simulink library "qss_tb_library"  (Simulink 10.0)
settings: Solver=ode45  StartTime=0.0  StopTime=1220  RelTol=1e-3
undefined symbols (not defined in the file): automatic_gearbox, cc_done, delta_h_C_air, DiscIntNeverNeededParam, dw_GG_c, eta_EG_map, eta_EM_map, eta_ice, g, h, H_o_m, H_u, i_FC_in, i_FC_max, k1, k2, k3, k4, k_cs, M_air, manual_gearbox, P_aux, P_CE_cutoff, P_CE_idle, P_CE_recup, P_CVT_opt, Q_BT_min, Q_SC_IC, r, rho, rho_f, t_c, T_CE_cutoff, T_CE_max, T_EG_c, T_EG_max, T_EM_max, theta_CE, theta_EM, V_CE_map, V_FC_out, w_CE_idle, w_CE_max, w_CE_upper, w_CVT_opt, w_EG_row, w_EG_upper, w_EM_row, w_EM_upper, w_GG_c
(part 1 of 4)
settings Model: Creator=buehli  LastModifiedBy=barka  ModifiedComment=rickardarvidsson -- Wed Jul 11 10:39:34 2018 -- Version 1.277  ExtModeAutoUpdateStatusClock=off
settings Model: ModifiedHistory=|
  | rickardarvidsson -- Wed Jul 11 10:39:34 2018 -- Version 1.277
  | 
  | rickardarvidsson -- Wed Jul 11 10:39:34 2018 -- Version 1.277
  | 
  | rickardarvidsson -- Wed Jul 11 10:39:21 2018 -- Version 1.276
  | 
  | rickardarvidsson -- Wed Jul 11 10:39:08 2018 -- Version 1.275
  | 
  | 2018b:
  | Updated Energy Buffer Libraries with 48V, HEV, PHEV, BEV Batteries.
  | Resistance, energy and current values adjusted for each cell type

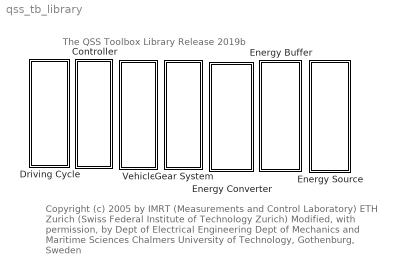
== system qss_tb_library ==
  note: Copyright (c) 2005 by IMRT (Measurements and Control Laboratory)
      | ETH Zurich (Swiss Federal Institute of Technology Zurich)
      |
      | Modified, with permission, by
      | Dept of Electrical Engineering
      | Dept of Mechanics and Maritime Sciences
      | Chalmers University of Technology, Gothenburg, Sweden
  note: The QSS Toolbox Library Release 2019b
  Controller : Subsystem
      mask Display: disp('Controller')
  Driving Cycle : Subsystem
      mask Display: disp('Driving Cycle')
  Energy Buffer : Subsystem
      mask Display: disp('Energy Buffer')
  Energy Converter : Subsystem
      mask Display: disp('Energy Converter')
  Energy Source : Subsystem
      mask Display: disp('Energy Source')
  Gear System : Subsystem
      mask Display: disp('Gear System')
  Vehicle : Subsystem
      mask Display: disp('Vehicle')

== system qss_tb_library/Controller ==
  Battery Controller : Subsystem  mask(Battery Controller){}
      mask help:
      | Control strategy (very primitive):
      | ========================
      | As soon as battery charge drops below level Q_BT_min, the CE/Generator
      | are started and operated at given load/speed for a fixed time period.
      | This time has been selected to guarantee the same battery level at the
      | end of the cycle.
      mask init:
      | init_BT_ctrl;
  CVT Controller : Subsystem  Tag=cvt controller  mask(CVT Controller){j_CVT_min=3, j_CVT_max=15, w_wheel_min=3, w_CVT_idle=100, w_CVT_upper=300}
      mask prompts: j_CVT_min "Lower gear ratio limit [-]"; j_CVT_max "Upper gear ratio limit [-]"; w_wheel_min "Minimum wheel speed [rad/s]"; w_CVT_idle "CVT idle speed [rad/s]"; w_CVT_upper "Maximum CVT speed [rad/s]"
      mask help:
      | This block calculates the optimum gear ratio and its change during one integration step for a CVT.
      |
      | Input:
      | =====
      | 	v	Speed [m/s]
      | 	dv_dt	Acceleration [m/s^2]
      |
      | Output:
      | ======
      | 	v_delay	Speed one step delayed [m/s]
      | 	dv_dt_delay	Acceleration one step delayed [m/s^2]
      | 	j_CVT	Gear ratio [-]
      | 	dj_CVT	Change of gear ratio [1/s]
      mask init:
      | init_CVT_ctrl;
  Control Unit (empty template) : Subsystem  Tag=control unit  mask(Control Unit){}
      mask help:
      | This block gives the user the opportunity to design his/her own control unit.
      |
      | The user can define the inputs and outputs  by himself/herself.
  "Hybrid Controller Unit  (Parallel, empty)" : Subsystem  mask(Hybrid Controller Unit){}
      mask help: Design your control strategy in this block.
      mask init:
      | init_HCU_parallel;

== system qss_tb_library/Driving Cycle ==
  Driving Cycle : Subsystem  Tag=cycle  mask(Driving Cycle){cyclename1=NEDC, stepsize=1, autostop=on}
      mask prompts: cyclename1 "Choose a cycle"; stepsize "Step size [s]"; autostop "Enable automatic simulation stop"
      mask help:
      | This block loads the cycle data such as time, speed, acceleration and gear number,  from the specified data file and makes it available on the output of the cycle block.
      |
      | Output:
      | ======
      | 	v	Speed [m/s]
      | 	a	Acceleration [m/s^2]
      | 	i	Gear number [-]
      | 	x_tot	Total distance [m]
      |
      | Tip:
      | ===
      | Probably you don't need the gear number "i". If so you can terminate
      | it with a "Terminator" out of the "Simulink Library/Connections."
      |
      | Driving cycle:
      | ===
      | Select a driving cycle from the list below or specify your own (place your .mat file in the
      | directory Data/DrivingCycles/UserDefined)
      |
      | ECE_MAN
      | ECE_R15s
      | EUDC
      | EUDC_MAN
      | City
      | City_MAN
      | NEDC
      | NEDC_MANl
      | GOT1
      | GOT2
      | GOT3
      | 10_15_MODE
      | 10_MODE
      | 10_MODE_3
      | 11_MODE
      | 11_MODE_4
      | 15_MODE
      | City_I
      | City_II
      | FTP_75
      | FTP_Highway
      |
      | WLTC
      | RTS95
      |
      |
      | Step size:
      | ========
      | Default value is 1. Don't change it, unless you are familiar with the programs of the QSS TB.
      |
      | Enable automatic simulation stop:
      | ===========================
      | Stops the simulation automatically at the end of the cycle.
      | Be careful: If you have a component in your model that has to run after the cycle has finished, e.g. a battery to charge, remove the mark!
      mask init:
      | init_driving_cycle1;
      mask Display: plot(T_zplot, V_zplot);
  Driving Cycle  (with performance  test possibility) : Subsystem  Tag=cycle  mask(Driving Cycle){cyclenr=Europe: NEDC, stepsize=1, autostop=on, test=off, v_init=0, v_end=0, acc_constant=0, gearon=[10 25 40 70], gearoff=[5 15 30 50]}
      mask prompts: cyclenr "Choose a cycle"; stepsize "Step size [s]"; autostop "Enable automatic simulation stop"; test "Acceleration performance test"; v_init "Start velocity [km/h]"; v_end "End velocity [km/h]"; acc_constant "Constant acceleration [m/s2]"; gearon "Switching points for upshift [km/h]"; gearoff "Switching points for downshift [km/h]"
      mask help:
      | This block loads the cycle data such as time, speed, acceleration and gear number,  from the specified data file and makes it available on the output of the cycle block.
      |
      | Output:
      | ======
      | 	v	Speed [m/s]
      | 	a	Acceleration [m/s^2]
      | 	i	Gear number [-]
      | 	x_tot	Total distance [m]
      |
      | Tip:
      | ===
      | Probably you don't need the gear number "i". If so you can terminate
      | it with a "Terminator" out of the "Simulink Library/Connections."
      |
      | Step size:
      | ========
      | Default value is 1. Don't change it, unless you are familiar with the programs of the QSS TB.
      |
      | Enable automatic simulation stop:
      | ===========================
      | Stops the simulation automatically at the end of the cycle.
      | Be careful: If you have a component in your model that has to run after the cycle has finished, e.g. a battery to charge, remove the mark!
      |
      | Acceleration Performance Test:
      | ===========================
      | This option will perform an acceleration test using a constant acceleration, from
      | start velocity to end velocity.
      | Gear shifting occuring to shifting schedule, defined by the user.
      mask init:
      | init_driving_cycle;
      mask TypeOptions cyclenr: Europe: ECE manual | Europe: ECE R15 spez | Europe: ECE R15 | Europe: EUDC | Europe: EUDC manual | Europe: City | Europe: City manual | Europe: NEDC | Europe: NEDC manual | Europe: GOT1 | Europe: GOT2 | Europe: GOT3 | Japan:  10-15-Mode | Japan:  10-Mode | Japan:  10-Mode-3 | Japan:  11-Mode | Japan:  11-Mode-4 | Japan:  15-Mode | USA:    City-I | USA:    City-II | USA:    FTP-75 | USA:    FTP-Highway
      mask Display: plot(T_zplot, V_zplot);
  Driving Cycle (no gradient) : Subsystem  Tag=cycle  mask(Driving Cycle){cyclename1=NEDC, stepsize=1, autostop=on}
      mask prompts: cyclename1 "Choose a cycle"; stepsize "Step size [s]"; autostop "Enable automatic simulation stop"
      mask help:
      | This block loads the cycle data such as time, speed, acceleration and gear number,  from the specified data file and makes it available on the output of the cycle block.
      |
      | Output:
      | ======
      | 	v	Speed [m/s]
      | 	a	Acceleration [m/s^2]
      | 	i	Gear number [-]
      | 	x_tot	Total distance [m]
      |
      | Tip:
      | ===
      | Probably you don't need the gear number "i". If so you can terminate
      | it with a "Terminator" out of the "Simulink Library/Connections."
      |
      | Driving cycle:
      | ===
      | Select a driving cycle from the list below or specify your own (place your .mat file in the
      | directory Data/DrivingCycles/UserDefined)
      |
      | ECE_MAN
      | ECE_R15s
      | EUDC
      | EUDC_MAN
      | City
      | City_MAN
      | NEDC
      | NEDC_MANl
      | GOT1
      | GOT2
      | GOT3
      | 10_15_MODE
      | 10_MODE
      | 10_MODE_3
      | 11_MODE
      | 11_MODE_4
      | 15_MODE
      | City_I
      | City_II
      | FTP_75
      | FTP_Highway
      |
      |
      | Step size:
      | ========
      | Default value is 1. Don't change it, unless you are familiar with the programs of the QSS TB.
      |
      | Enable automatic simulation stop:
      | ===========================
      | Stops the simulation automatically at the end of the cycle.
      | Be careful: If you have a component in your model that has to run after the cycle has finished, e.g. a battery to charge, remove the mark!
      mask init:
      | init_driving_cycle1;
      mask Display: plot(T_zplot, V_zplot);

== system qss_tb_library/Energy Buffer ==
  note: Batteries for hybrid vehicles
  48V Battery : Subsystem  Tag=battery  mask(Battery){cell_series=14, cell_parallel=1, Q_BT_IC_rel=50}
      mask prompts: cell_series "Number of series cells"; cell_parallel "Number  of parallel cells"; Q_BT_IC_rel "Initial charge of battery [%]"
      mask help:
      | This block simulates a 48 V battery.
      | The open circuit voltage and resistance depend on the battery state of charge.
      | Open circuit voltage is dependent on how many batteries that are connected in series
      | Each cell has a capacity of 8 Ah and the cell open-circuit voltage is 3.8 V at 50% SoC.
      | The maximum peak current output per each cell is +/- 400 A.
      |
      | This type of battery cell has a significant reduction of power below 20% SoC
      |
      | Input:
      | =====
      | 	P_BT	Power from/to the battery [W]
      | 		P_BT < 0: battery charging
      | 		P_BT > 0: battery discharging
      | 	x_tot	Total distance [m]
      |
      | Output:
      | ======
      | 	B_SoC	State of charge ratio [-]
      | 	U_BT	Voltage of the battery [V]
      | 	E_BT	Energy consumption [kWh/100 km]
      mask init:
      | init_BT_Assign;
  BEV Battery : Subsystem  Tag=battery  mask(Battery){cell_series=100, cell_parallel=2, Q_BT_IC_rel=50}
      mask prompts: cell_series "Number of series cells"; cell_parallel "Number  of parallel cells"; Q_BT_IC_rel "Initial charge of battery [%]"
      mask help:
      | This block simulates a battery.
      | The open circuit voltage and resistance depend on the battery state of charge.
      | Open circuit voltage is dependent on how many batteries that are connected in series
      | Each cell has a capacity of 96 Ah and the cell open-circuit voltage is 3.8 V at 50% SoC which means that each cell can provide from 360 Wh of energy depending on the discharge current
      | Max peak current is set to +/- 120 A per cell
      |
      | Input:
      | =====
      | 	P_BT	Power from/to the battery [W]
      | 		P_BT < 0: battery charging
      | 		P_BT > 0: battery discharging
      | 	x_tot	Total distance [m]
      |
      | Output:
      | ======
      | 	B_SoC	State of charge ratio [-]
      | 	U_BT	Voltage of the battery [V]
      | 	E_BT	Energy consumption [kWh/100 km]
      mask init:
      | init_BT_Assign;
  Battery Assignment : Subsystem  Tag=battery  mask(Battery){cell_series=80, cell_parallel=3, Q_BT_IC_rel=50}
      mask prompts: cell_series "Number of series cells"; cell_parallel "Number  of parallel cells"; Q_BT_IC_rel "Initial charge of battery [%]"
      mask help:
      | This block simulates a battery.
      | The open circuit voltage and resistance depend on the battery state of charge.
      | The battery voltage is depending on how many cells which are connected in series.
      | Each cell has a capacity of 54 Ah and the cell open-circuit voltage is 3.8 V at 50% SoC which means that each cell can store about 205 Wh of energy.
      |
      | This type of battery cell has a significant reduction of power below 20% SoC
      |
      | Input:
      | =====
      | 	P_BT	Power from/to the battery [W]
      | 		P_BT < 0: battery charging
      | 		P_BT > 0: battery discharging
      | 	x_tot	Total distance [m]
      |
      | Output:
      | ======
      | 	B_SoC	State of charge ratio [-]
      | 	U_BT	Voltage of the battery [V]
      | 	E_BT	Energy consumption [kWh/100 km]
      mask init:
      | init_BT_Assign;
  HEV Battery : Subsystem  Tag=battery  mask(Battery){cell_series=80, cell_parallel=1, Q_BT_IC_rel=50}
      mask prompts: cell_series "Number of series cells"; cell_parallel "Number  of parallel cells"; Q_BT_IC_rel "Initial charge of battery [%]"
      mask help:
      | This block simulates a HEV battery.
      | The open circuit voltage and resistance depend on the battery state of charge.
      | Open circuit voltage is dependent on how many batteries that are connected in series
      | Each cell has a capacity of 15 Ah and the cell open-circuit voltage is 3.8 V at 50% SoC.
      | Max peak power output is +/- 100 A for each cell
      |
      | Input:
      | =====
      | 	P_BT	Power from/to the battery [W]
      | 		P_BT < 0: battery charging
      | 		P_BT > 0: battery discharging
      | 	x_tot	Total distance [m]
      |
      | Output:
      | ======
      | 	B_SoC	State of charge ratio [-]
      | 	U_BT	Voltage of the battery [V]
      | 	E_BT	Energy consumption [kWh/100 km]
      mask init:
      | init_BT_Assign;
  PHEV Battery : Subsystem  Tag=battery  mask(Battery){cell_series=100, cell_parallel=1, Q_BT_IC_rel=50}
      mask prompts: cell_series "Number of series cells"; cell_parallel "Number  of parallel cells"; Q_BT_IC_rel "Initial charge of battery [%]"
      mask help:
      | This block simulates a PHEV battery.
      | The open circuit voltage and resistance depend on the battery state of charge.
      | Open circuit voltage is dependent on how many batteries that are connected in series
      | Each cell has a capacity of 35 Ah and the cell open-circuit voltage is 3.8 V at 50% SoC.
      | Max peak current per cell is +/- 200 A
      |
      | Input:
      | =====
      | 	P_BT	Power from/to the battery [W]
      | 		P_BT < 0: battery charging
      | 		P_BT > 0: battery discharging
      | 	x_tot	Total distance [m]
      |
      | Output:
      | ======
      | 	B_SoC	State of charge ratio [-]
      | 	U_BT	Voltage of the battery [V]
      | 	E_BT	Energy consumption [kWh/100 km]
      mask init:
      | init_BT_Assign;
  Supercapacitor : Subsystem  Tag=supercap  mask(Supercapacitor){C_SC=8, R_SC=0.72, U_SC_max=225, P_SC_max=17500, Q_SC_IC_rel=95, N_SC=6}
      mask prompts: C_SC "Capacity of each supercap [F]"; R_SC "Internal resistance of each supercap [Ohm]"; U_SC_max "Maximum voltage of each supercap  [V]"; P_SC_max "Maximum power of each supercap [W]"; Q_SC_IC_rel "Initial charge of each supercap [%]"; N_SC "Number of supercaps (parallel connection) [-]"
      mask help:
      | The supercap is a fast electric energy buffer.
      |
      | Input:
      | =====
      | 	P_SC	Power to/from the supercap [W]
      | 		P_SC < 0: SC charging
      | 		P_SC > 0: SC discharging
      |
      | Output:
      | ======
      | 	U_SC	Voltage of the supercap [V]
      mask init:
      | init_SC;

== system qss_tb_library/Energy Converter ==
  CE Assignment : Subsystem  Tag=combustion engine  mask(Combustion Engine (based on consumption map)){engine_type=Gasoline, P_ice=100, ENABLE_FUEL_CUTOFF=off}
      mask prompts: engine_type "Engine type"; P_ice "Power [kW]"; ENABLE_FUEL_CUTOFF "Enable fuel cutoff"
      mask help:
      | This block simulates the behaviour of a combustion engine. The block is based on consumption maps for medium sized passenger cars.
      |
      | NA Gasoline:
      | max power @ 5000 rpm
      | max torque @ 3000 rpm
      |
      | Small Diesel:
      | max power @ 4500 rpm
      | max torque @ 2000 rpm
      |
      | Large Diesel:
      | max power @ 1500 rpm
      | max torque @ 1500 rpm
      |
      |
      | Input:
      | =====
      | 	w_gear	Speed of the fly wheel [rad/s]
      | 	dw_dt_gear	Acceleration of the fly wheel [rad/s^2]
      | 	T_gear	Torque on the fly wheel [Nm]
      |
      | Output:
      | ======
      | 	P_CE	Fuel power consumed by the combustion engine [W]
      mask init:
      | init_AssCE_map;
      mask TypeOptions engine_type: Gasoline | Small Diesel | Large Diesel
  Combustion Engine (Willans-approximation  with overload detection) : Subsystem  Tag=combustion engine  mask(Combustion Engine (based on Willans approximation)){engine_type=Otto, V_d=0.708, theta_CE=0.05, S=50, B=45, maxTorque=[177 4300], maxPower=[96 6100], w_CE_upper=700, w_CE_idle=105, P_CE_idle=2600, P_aux=300, e=0.46, PI=2, p_me0g=1, ENABLE_FUEL_CUTOFF=on, T_CE_cutoff=5, P_CE_cutoff=0}
      mask prompts: engine_type "Engine type"; V_d "Displacement [l]"; theta_CE "Engine inertia [kg*m^2]"; S "Stroke [mm]"; B "Bore diameter [mm]"; maxTorque "Max torque @ rpm [Nm rpm]"; maxPower "Max Power @ rpm [kW rpm]"; w_CE_upper "Maximum engine speed [rad/s]"; w_CE_idle "Engine speed at idle [rad/s]"; P_CE_idle "Engine power at idle [W]"; P_aux "Power required by auxiliaries  [W]"; e "1. Willans parameter: Engine internal thermodynamic efficiency [-]"; PI "2. Willans parameter: Maximum boost ratio [-]"; p_me0g "3. Willans parameter: Gas exchange losses [bar]"; ENABLE_FUEL_CUTOFF "Enable fuel cutoff"; T_CE_cutoff "Engine torque at fuel cutoff [Nm]"; P_CE_cutoff "Power at fuel cutoff [W]"
      mask help:
      | This block simulates the behaviour of a combustion engine. The block is based on the Willans approximation with friction part based on the ETH model. The model has been extended with overload and overspeed  detection.
      |
      | Input:
      | =====
      | 	w_gear		Speed of the fly wheel [rad/s]
      | 	dw_gear	Acceleration of the fly wheel [rad/s^2]
      | 	T_gear		Torque on the fly wheel [Nm]
      |
      | Output:
      | ======
      | 	P_CE		Power produced by the combustion engine [W]
      mask init:
      | init_CE_willans2;
      mask TypeOptions engine_type: Otto | Diesel
  Combustion Engine (Willans-approximation) : Subsystem  Tag=combustion engine  mask(Combustion Engine (based on Willans approximation)){engine_type=Otto, V_d=0.708, theta_CE=0.05, S=50, B=45, w_CE_idle=105, P_CE_idle=2600, P_aux=300, e=0.46, PI=2, p_me0g=1, ENABLE_FUEL_CUTOFF=on, T_CE_cutoff=5, P_CE_cutoff=0}
      mask prompts: engine_type "Engine type"; V_d "Displacement [l]"; theta_CE "Engine inertia [kg*m^2]"; S "Stroke [mm]"; B "Bore diameter [mm]"; w_CE_idle "Engine speed at idle [rad/s]"; P_CE_idle "Engine power at idle [W]"; P_aux "Power required by auxiliaries  [W]"; e "1. Willans parameter: Engine internal thermodynamic efficiency [-]"; PI "2. Willans parameter: Maximum boost ratio [-]"; p_me0g "3. Willans parameter: Gas exchange losses [bar]"; ENABLE_FUEL_CUTOFF "Enable fuel cutoff"; T_CE_cutoff "Engine torque at fuel cutoff [Nm]"; P_CE_cutoff "Power at fuel cutoff [W]"
      mask help:
      | This block simulates the behaviour of a combustion engine. The block is based on the Willans approximation with friction part based on the ETH model.
      |
      | Input:
      | =====
      | 	w_gear		Speed of the fly wheel [rad/s]
      | 	dw_gear	Acceleration of the fly wheel [rad/s^2]
      | 	T_gear		Torque on the fly wheel [Nm]
      |
      | Output:
      | ======
      | 	P_CE		Power produced by the combustion engine [W]
      mask init:
      | init_CE_willans;
      mask TypeOptions engine_type: Otto | Diesel
  Combustion Engine (consumption map) : Subsystem  Tag=combustion engine  mask(Combustion Engine (based on consumption map)){engine_type=Otto, mapname='qss_ce_original_map', V_d=0.708, scale_CE=1, theta_CE=0.05, w_CE_idle=105, P_CE_idle=2600, P_aux=300, ENABLE_FUEL_CUTOFF=on, T_CE_cutoff=5, P_CE_cutoff=0}
      mask prompts: engine_type "Engine type"; mapname "Consumption map name"; V_d "Displacement [l]"; scale_CE "Engine scaling factor [-]"; theta_CE "Engine inertia [kg*m^2]"; w_CE_idle "Engine speed at idle [rad/s]"; P_CE_idle "Engine power at idle [W]"; P_aux "Power required by auxiliaries [W]"; ENABLE_FUEL_CUTOFF "Enable fuel cutoff"; T_CE_cutoff "Engine torque at fuel cutoff [Nm]"; P_CE_cutoff "Power at fuel cutoff [W]"
      mask help:
      | This block simulates the behaviour of a combustion engine. The block is based on a consumption map. The map is located in the Data/EnergyConverter/CombustionEngine directory.
      |
      | Input:
      | =====
      | 	w_gear		Speed of the fly wheel [rad/s]
      | 	dw_gear	Acceleration of the fly wheel [rad/s^2]
      | 	T_gear		Torque on the fly wheel [Nm]
      |
      | Output:
      | ======
      | 	P_CE		Power produced by the combustion engine [W]
      |
      | Consumption map:
      | ======
      |
      | The consumption map file must contain the following variables:
      |
      | V_CE_map		% Consumption map 			[kg/s]
      | eta_CE_map                       % Efficiency map                            		[-]
      | w_CE_row                         % Engine speed range                       		[rad/s]
      | p_me_col                            % Brake mean effective pressure range       	[Pa]
      | w_CE_max                         % Maximum engine speed                     		[rad/s]
      | p_me_max                          % Maximum brake mean effective pressure     	[Pa]
      mask init:
      | init_CE_map;
      mask TypeOptions engine_type: Otto | Diesel
  Combustion Engine (ideal) : Subsystem  Tag=combustion engine  mask(Combustion Engine (ideal)){engine_type=Otto, theta_CE=0.05, P_aux=0, recuperation=No_recuperation, idling=off, idle_power=2600}
      mask prompts: engine_type "Engine type"; theta_CE "Engine inertia [kg*m^2]"; P_aux "Power required by auxiliaries [W]"; recuperation "Recuperation of energy"; idling "Idling power consumption"; idle_power "Idling power consumption [W]"
      mask help:
      | This block simulates the behaviour of a combustion engine. The block is based on an ideal power supply. If engine type ideal is selected then the engine efficiency is 1, else it is 0.4 for otto and 0.5 for diesel.
      |
      | Input:
      | =====
      | 	w_gear		Speed of the fly wheel [rad/s]
      | 	dw_gear	Acceleration of the fly wheel [rad/s^2]
      | 	T_gear		Torque on the fly wheel [Nm]
      |
      | Output:
      | ======
      | 	P_CE		Power produced by the combustion engine [W]
      mask init:
      | init_CE_ideal;
      mask TypeOptions engine_type: Otto | Diesel
      mask TypeOptions recuperation: No_recuperation | Perfect_recuperation
  EG Assignment : Subsystem  mask(Electric Generator){P_eg=30}
      mask prompts: P_eg "Maximum mechanical power [kW]"
      mask help:
      | This block simulates the behaviour of an electric generator. The block is based on an efficiency map.
      |
      | Input:
      | =====
      | 	w_gear	Speed of the generator [rad/s]
      | 	T_gear	Torque of the generator [Nm]
      |
      | Output:
      | ======
      | 	P_EG	Electric power of the generator [W]
      |
      | Generator map:
      | ======
      | The generator map file must contain the following variables:
      | eta_EG_map		% Efficiency map                    [-]
      | w_EG_row                        % Generator speed range             [rad/s]
      | T_EG_col		% Generator torque range            [Nm]
      | w_EG_max		% Maximum generator speed           [rad/s]
      | T_EG_max		% Maximum generator torque          [Nm]
      |
      | ======
      mask init:
      | init_EG_ass;
  EM Assignment : Subsystem  mask(Electric Motor){P_em=100}
      mask prompts: P_em "Power [kW]"
      mask help:
      | This block simulates the behaviour of an electric motor. The block is based on an efficiency map. The map is located in the Data/EnergyConvertter/ElectricMotor directory.
      |
      | Maximum speed och the electric motor is 6000 rpm
      | Field weakening region starts at 1500 rpm
      | Maximum mechanical power is at 2150 rpm
      | The maximum torque is 5.98 Nm/kW multiplied with the power you select.
      |
      | Input:
      | =====
      | 	w_gear	Speed of the motor [rad/s]
      | 	dw_dt_gear	Acceleration of the motor [rad/s^2]
      | 	T_gear	Torque of the motor [Nm]
      |
      | Output:
      | ======
      | 	P_EM	Electric Power consumed by the  motor [W]
      mask init:
      | init_EM_ass;
  Electric Generator : Subsystem  mask(Electric Generator){egmapname='qss_eg_original_map', scale_EG=1}
      mask prompts: egmapname "Generator map name"; scale_EG "Generator scaling factor [-]"
      mask help:
      | This block simulates the behaviour of an electric generator. The block is based on an efficiency map.
      |
      | Input:
      | =====
      | 	w_gear		Speed of the fly wheel [rad/s]
      | 	T_gear		Torque on the fly wheel [Nm]
      |
      | Output:
      | ======
      | 	P_EG		Power of the electric generator [W]
      |
      | Generator map:
      | ======
      | The generator map file must contain the following variables:
      | eta_EG_map		% Efficiency map                    [-]
      | w_EG_row                        % Generator speed range             [rad/s]
      | T_EG_col		% Generator torque range            [Nm]
      | w_EG_max		% Maximum generator speed           [rad/s]
      | T_EG_max		% Maximum generator torque          [Nm]
      mask init:
      | init_EG;
  Electric Motor : Subsystem  mask(Electric Motor){emmapname='qss_em_original_map', scale_EM=1, theta_EM=0.1, P_aux=0}
      mask prompts: emmapname "Motor map name"; scale_EM "Motor scaling factor [-]"; theta_EM "Motor inertia [kg*m2]"; P_aux "Power required by auxiliaries [W]"
      mask help:
      | This block simulates the behaviour of an electric motor. The block is based on an efficiency map. The map is located in the Data/EnergyConvertter/ElectricMotor directory.
      |
      | Input:
      | =====
      | 	w_gear		Speed of the fly wheel [rad/s]
      | 	dw_gear	Acceleration of the fly wheel [rad/s^2]
      | 	T_gear		Torque on the fly wheel [Nm]
      |
      | Output:
      | ======
      | 	P_EM		Power produced by the electric motor [W]
      |
      | Motor map:
      | ======
      | The motor map file must contain the following variables:
      | eta_EM_map		% Efficiency map                [-]
      | w_EM_row		% Motor speed range             [rad/s]
      | T_EM_col		% Motor torque range            [Nm]
      | w_EM_max		% Maximum motor speed           [rad/s]
      | load T_EM_max	% Maximum motor torque          [Nm]
      mask init:
      | init_EM;
  Fuel Cell : Subsystem  Tag=fuelcell  mask(Fuel Cell){N_FC=880, A_FC=190 * 1e4, V_th=1.2, P_FC_idle=2000, eta_EM_C=0.75, eta_C=0.7, pi_C=1.3, T_air=25, l_air=1.5}
      mask prompts: N_FC "Number of fuel cells per stack (series connection) [-]"; A_FC "Size of fuel cell [m^2]"; V_th "Theoretical fuel cell voltage [V]"; P_FC_idle "Idle power [W]"; eta_EM_C "E-motor for air compressor efficiency [-]"; eta_C "Air compressor efficiency [-]"; pi_C "Air compression ratio [-]"; T_air "Air temperature [°C]"; l_air "Air to fuel ratio [-]"
      mask help:
      | This block simulates a fuel cell and converts fuel into electric energy.
      |
      | Input:
      | =====
      | 	P_in		Power required by the fuel cell [W]
      |
      | Output:
      | ======
      | 	P_FC		Power produced by the fuel cell [W]
      mask init:
      | init_FC;

== system qss_tb_library/Energy Source ==
  Display : Display
  Tank : Subsystem  Tag=tank  mask(Tank){fuel=Gasoline, flag_cold_start=on}
      mask prompts: flag_cold_start "Include cold start losses"
      mask help:
      | This block integrates the power (the fuel mass flow) required by the combustion engine or the fuel cell and calculates the energy consumption in liter/100 km.
      |
      | Input:
      | =====
      | 	P_fuel	Power (fuel mass flow) required [W]
      | 	x_tot	Total distance [m]
      |
      | Output:
      | ======
      | 	V	Fuel consumption [liter/100 km]
      mask init:
      | init_tank;
      mask TypeOptions fuel: Gasoline | Diesel | Hydrogen
  wires:
  Tank/1(liter/100 km) -> Display/1

== system qss_tb_library/Gear System ==
  note: Main blocks to use in course
  Automatic Gear Box : Subsystem  Tag=transmission  mask(Automatic Gear Box){nog=5, i=[3.38 1.76 1.12 0.89 0.7], i_diff=4.45, gearon=[10 25 40 70], gearoff=[2 15 30 50], d=0.62, e_GT=0.98, P_GT0=300, w_wheel_min=1}
      mask prompts: nog "Number of gears"; i "Gear ratio vector"; i_diff "Differential gear [-]"; gearon "Switching points for upshift [km/h]"; gearoff "Switching points for downshift [km/h]"; d "Wheel diameter"; e_GT "Efficiency [-]"; P_GT0 "Idling losses (friction) [W]"; w_wheel_min "Minimum wheel speed beyond which losses are generated [rad/s]"
      mask help:
      | This block simulates a automatic gear box, can handle up to 16 gears.
      |
      | Input:
      | =====
      | 	w_wheel	Speed of the wheel [rad/s]
      | 	dw_dt_wheel	Acceleration of the wheel [rad/s^2],
      | 	T_wheel	Torque on the wheel [Nm]
      | 	i	Gear number [-]
      |
      | Output:
      | ======
      | 	w_MGB	Speed of the fly wheel [rad/s]
      | 	dw_dt_MGB	Acceleration of the fly wheel [rad/s^2]
      | 	T_MGB	Torque on the fly wheel [Nm]
      |
      | Number of gears:
      | ======
      | Specify the number of forward gears
      |
      | Shifting points for upshift:
      | ======
      | Vector specifying the velocity for shifting
      | [first_to_second_gear    second_to_third_gear    ....]
      | The number of elements in the vector should be Number of gears - 1.
      |
      | Shifting points for udownshift:
      | ======
      | Simular to upshift
      | [second_to_first_gear    third_to_second_gear    ....]
      mask init:
      | init_AGB;
  Continuously Variable Transmission : Subsystem  Tag=cvt  mask(CVT){e_CVT=0.97, P_CVT0=400, w_wheel_min=3}
      mask prompts: e_CVT "Efficiency [-]"; P_CVT0 "Idling losses (friction) [W]"; w_wheel_min "Minimum wheel speed beyond which losses are generated [rad/s]"
      mask help:
      | This block simulates a CVT transmission.
      |
      | Input:
      | =====
      | 	w_wheel	Speed of the wheel [rad/s]
      | 	dw_dt_wheel	Acceleration of the wheel [rad/s^2],
      | 	T_wheel	Torque on the wheel [Nm]
      | 	j_CVT	Gear ratio [-]
      | 	dj_CVT	Change of gear ratio [1/s]
      |
      | Output:
      | ======
      | 	w_CVT	Speed of the fly wheel [rad/s]
      | 	dw_dt_CVT	Acceleration of the fly wheel [rad/s^2]
      | 	T_CVT	Torque on the fly wheel [Nm]
      mask init:
      | init_CVT;
  Manual Gear Box : Subsystem  Tag=transmission  mask(Manual Gear Box){i_1=3.38, i_2=1.76, i_3=1.12, i_4=0.89, i_5=0.7, i_diff=4.45, e_GT=0.98, P_GT0=300, w_wheel_min=1}
      mask prompts: i_1 "1. gear [-]"; i_2 "2. gear [-]"; i_3 "3. gear [-]"; i_4 "4. gear [-]"; i_5 "5. gear [-]"; i_diff "Differential gear [-]"; e_GT "Efficiency [-]"; P_GT0 "Idling losses (friction) [W]"; w_wheel_min "Minimum wheel speed beyond which losses are generated [rad/s]"
      mask help:
      | This block simulates a manual gear box.
      |
      | Input:
      | =====
      | 	w_wheel	Speed of the wheel [rad/s]
      | 	dw_dt_wheel	Acceleration of the wheel [rad/s^2],
      | 	T_wheel	Torque on the wheel [Nm]
      | 	i	Gear number [-]
      |
      | Output:
      | ======
      | 	w_MGB	Speed of the fly wheel [rad/s]
      | 	dw_dt_MGB	Acceleration of the fly wheel [rad/s^2]
      | 	T_MGB	Torque on the fly wheel [Nm]
      mask init:
      | init_MGB;
  Simple Transmission : Subsystem  Tag=simple transmission  mask(Simple Transmission){gear_ratio=2, e_GT=0.98, P_GT0=50, w_wheel_min=1}
      mask prompts: gear_ratio "Gear ratio [-]"; e_GT "Efficiency [-]"; P_GT0 "Idling losses (friction) [W]"; w_wheel_min "Minimum wheel speed beyond which losses are generated [rad/s]"
      mask help:
      | This block simulates a transmission with a fixed gear ratio.
      |
      | Input:
      | =====
      | 	w_wheel	Speed of the wheel [rad/s]
      | 	dw_dt_wheel	Acceleration of the wheel [rad/s^2]
      | 	T_wheel	Torque on the wheel [Nm]
      |
      | Output:
      | ======
      | 	w_trans	Speed of the fly wheel [rad/s]
      | 	dw_dt_trans	Acceleration of the fly wheel [rad/s^2]
      | 	T_trans	Torque on the fly wheel [Nm]
      mask init:
      | init_transmission;
  Simple Transmission2 : Subsystem  Tag=simple transmission  mask(Simple Transmission2){}
      mask help:
      | This block simulates an ideal transmission (no losses).
      |
      | Input:
      | =====
      | 	w_wheel	Speed of the wheel [rad/s]
      | 	dw_dt_wheel	Acceleration of the wheel [rad/s^2]
      | 	T_wheel	Torque on the wheel [Nm]
      |
      | Output:
      | ======
      | 	w_trans	Speed of the fly wheel [rad/s]
      | 	dw_dt_trans	Acceleration of the fly wheel [rad/s^2]
      | 	T_trans	Torque on the fly wheel [Nm]
      mask init:
      | init_transmission;

== system qss_tb_library/Vehicle ==
  Simple wheel model : Subsystem  Tag=simple transmission  mask(Simple wheel model){d_wheel=0.62}
      mask prompts: d_wheel "Wheel diameter [m]"
      mask help:
      | This block simulates a simple wheel model without tire slip and no losses.
      |
      | Input:
      | =====
      | 	v_veh	Speed of the vehicle [m/s]
      | 	a_veh	Acceleration of the vehicle [m/s^2]
      | 	F_Trac	Traction force [N]
      |
      | Output:
      | ======
      | 	w_wheel		Speed of the wheel shaft [rad/s]
      | 	dw_dt_wheel		Acceleration of the wheel shaft [rad/s^2]
      | 	T_wheel		Torque on the wheel shaft [Nm]
  Vehicle : Subsystem  Tag=vehicle  mask(Vehicle){m_f=1500, A_f=2.5, cw=0.30, mu=0.01, k_inertia=4}
      mask prompts: m_f "Total mass of the vehicle [kg]"; A_f "Vehicle cross section [m^2]"; cw "Drag coefficient [-]"; mu "Rolling resistance coefficient [-]"; k_inertia "Mass increase due to Rotating inertia [%]"
      mask help:
      | This block computes the force required by the vehicle.
      |
      | Input:
      | =====
      | 	v	Speed [m/s]
      | 	a	Acceleration [m/s^2]
      |    	alfa    	Road inclination angle [rad]
      |
      | Output:
      | ======
      | 	v_veh	Speed of the vehicle [m/s]
      | 	a_veh	Acceleration of the vehicle [m/s^2]
      | 	F_Trac	Traction Force required from the powertrain [N]
      mask init:
      | init_vehicle;

== system qss_tb_library/Controller/Battery Controller ==
  Q_BT : Inport
  Constant : Constant  OutDataTypeStr=boolean
  Constant1 : Constant  Value=Q_BT_min
  Constant2 : Constant  Value=0  OutDataTypeStr=boolean
  Demux : Demux  Outputs=3
  Geno-Group On : Subsystem
  S-R Flip-Flop : Subsystem
  Sum : Sum  Inputs=+-  SaturateOnIntegerOverflow=on  InputSameDT=on  OutDataTypeStr=Inherit: Same as first input
  Switch : Switch  SaturateOnIntegerOverflow=on  InputSameDT=on
  Terminator1 : Terminator
  To Workspace1 : ToWorkspace  VariableName=w_ctrl  SampleTime=-1
  To Workspace2 : ToWorkspace  VariableName=T_ctrl  SampleTime=-1
  To Workspace5 : ToWorkspace  VariableName=cc_on  SampleTime=-1
  w_ctrl : Outport  InitialOutput=0
  dw_dt_ctrl : Outport  Port=2  InitialOutput=0
  T_ctrl : Outport  Port=3  InitialOutput=0
  wires:
  S-R Flip-Flop/1(Q) -> To Workspace5/1, Geno-Group On/1(cc_on)
  Switch/1 -> S-R Flip-Flop/1(S)
  S-R Flip-Flop/2(!Q) -> Terminator1/1
  Geno-Group On/1(OutOn) -> Demux/1
  Demux/3 -> To Workspace2/1, T_ctrl/1
  Demux/2 -> dw_dt_ctrl/1
  Demux/1 -> To Workspace1/1, w_ctrl/1
  Geno-Group On/2(done) -> S-R Flip-Flop/2(R)
  Q_BT/1 -> Sum/1
  Sum/1 -> Switch/2
  Constant2/1 -> Switch/1
  Constant/1 -> Switch/3
  Constant1/1 -> Sum/2

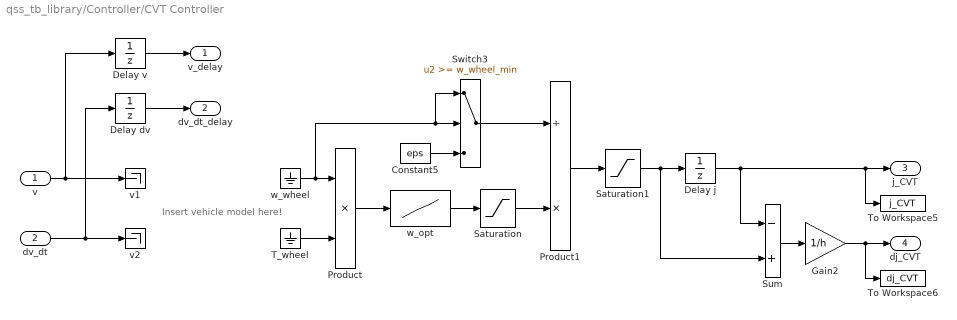
== system qss_tb_library/Controller/CVT Controller ==
  note: Insert vehicle
      | model here!
  v : Inport
  dv_dt : Inport  Port=2
  Constant5 : Constant  Value=eps
  Delay dv : UnitDelay  SampleTime=h  HasFrameUpgradeWarning=on
  Delay j : UnitDelay  InitialCondition=j_CVT_min  SampleTime=h  HasFrameUpgradeWarning=on
  Delay v : UnitDelay  SampleTime=h  HasFrameUpgradeWarning=on
  Gain2 : Gain  Gain=1/h  SaturateOnIntegerOverflow=on  OutDataTypeStr=Inherit: Same as input  ParamDataTypeStr=Inherit: Same as input
  Product : Product  SaturateOnIntegerOverflow=on  RndMeth=Zero  InputSameDT=on  OutDataTypeStr=Inherit: Same as first input
  Product1 : Product  Inputs=/*  SaturateOnIntegerOverflow=on  RndMeth=Zero  InputSameDT=on  OutDataTypeStr=Inherit: Same as first input
  Saturation : Saturate  UpperLimit=w_CVT_upper  LowerLimit=w_CVT_idle
  Saturation1 : Saturate  UpperLimit=j_CVT_max  LowerLimit=j_CVT_min
  Sum : Sum  Inputs=-+  SaturateOnIntegerOverflow=on  InputSameDT=on  OutDataTypeStr=Inherit: Same as first input
  Switch3 : Switch  Threshold=w_wheel_min  SaturateOnIntegerOverflow=on  InputSameDT=on
  T_wheel : Ground
  To Workspace5 : ToWorkspace  VariableName=j_CVT  SampleTime=-1
  To Workspace6 : ToWorkspace  VariableName=dj_CVT  SampleTime=-1
  v1 : Terminator
  v2 : Terminator
  w_opt : Lookup  InputValues=P_CVT_opt  Table=w_CVT_opt  SaturateOnIntegerOverflow=on
  w_wheel : Ground
  v_delay : Outport  InitialOutput=0
  dv_dt_delay : Outport  Port=2  InitialOutput=0
  j_CVT : Outport  Port=3  InitialOutput=0
  dj_CVT : Outport  Port=4  InitialOutput=0
  wires:
  Gain2/1 -> To Workspace6/1, dj_CVT/1
  T_wheel/1 -> Product/2
  Product1/1 -> Saturation1/1
  Saturation/1 -> Product1/2
  w_wheel/1 -> Switch3/2, Switch3/1, Product/1
  Constant5/1 -> Switch3/3
  dv_dt/1 -> Delay dv/1, v2/1
  v/1 -> Delay v/1, v1/1
  Delay dv/1 -> dv_dt_delay/1
  Switch3/1 -> Product1/1
  Delay j/1 -> To Workspace5/1, j_CVT/1, Sum/1
  Saturation1/1 -> Delay j/1, Sum/2
  Product/1 -> w_opt/1
  w_opt/1 -> Saturation/1
  Delay v/1 -> v_delay/1
  Sum/1 -> Gain2/1

== system qss_tb_library/Controller/Control Unit (empty template) ==
  note: Control Unit: custom designed
  y 1 : Inport
  y p : Inport  Port=2
  Ground : Ground
  Ground1 : Ground
  Terminator : Terminator
  Terminator1 : Terminator
  u 1 : Outport  InitialOutput=0
  u m : Outport  Port=2  InitialOutput=0
  wires:
  Ground/1 -> u 1/1
  Ground1/1 -> u m/1
  y 1/1 -> Terminator/1
  y p/1 -> Terminator1/1

== system qss_tb_library/Controller/Hybrid Controller Unit  (Parallel, empty) ==
  w_wheel : Inport
  dw_dt_wheel : Inport  Port=2
  T_wheel : Inport  Port=3
  Q_BT : Inport  Port=4
  w_ice : Outport  InitialOutput=0
  dw_dt_ice : Outport  Port=2  InitialOutput=0
  T_ice : Outport  Port=3  InitialOutput=0
  w_em : Outport  Port=4  InitialOutput=0
  dw_dt_em : Outport  Port=5  InitialOutput=0
  T_em : Outport  Port=6  InitialOutput=0

== system qss_tb_library/Driving Cycle/Driving Cycle ==
  note: Speed
  Clock : Clock
  Constant : Constant  Value=0
  Cycle data : FromWorkspace  VariableName=[T_z, V_z, D_z, G_z]  SampleTime=h
  Demux : Demux  Outputs=3
  Differentiation : Subsystem
  Integration : Subsystem
  Terminator : Terminator
  Time : Display
  To Workspace1 : ToWorkspace  VariableName=t  SampleTime=-1
  To Workspace2 : ToWorkspace  VariableName=x_tot  SampleTime=-1
  To Workspace3 : ToWorkspace  VariableName=alfa  SampleTime=-1
  To Workspace4 : ToWorkspace  VariableName=a  SampleTime=-1
  To Workspace5 : ToWorkspace  VariableName=v  SampleTime=-1
  To Workspace6 : ToWorkspace  VariableName=i  SampleTime=-1
  v : Outport  InitialOutput=0
  a : Outport  Port=2  InitialOutput=0
  alfa : Outport  Port=3  InitialOutput=0
  i : Outport  Port=4  InitialOutput=0
  x_tot : Outport  Port=5  InitialOutput=0
  wires:
  Constant/1 -> alfa/1, To Workspace3/1
  Clock/1 -> To Workspace1/1, Time/1
  Demux/3 -> To Workspace6/1, i/1  "Gear ratio"
  Integration/1(x_tot) -> To Workspace2/1, x_tot/1
  Demux/2 -> Terminator/1
  Differentiation/1(D_z) -> a/1, To Workspace4/1
  Cycle data/1 -> Demux/1
  Demux/1 -> To Workspace5/1, v/1, Differentiation/1(V_z), Integration/1(V_z)

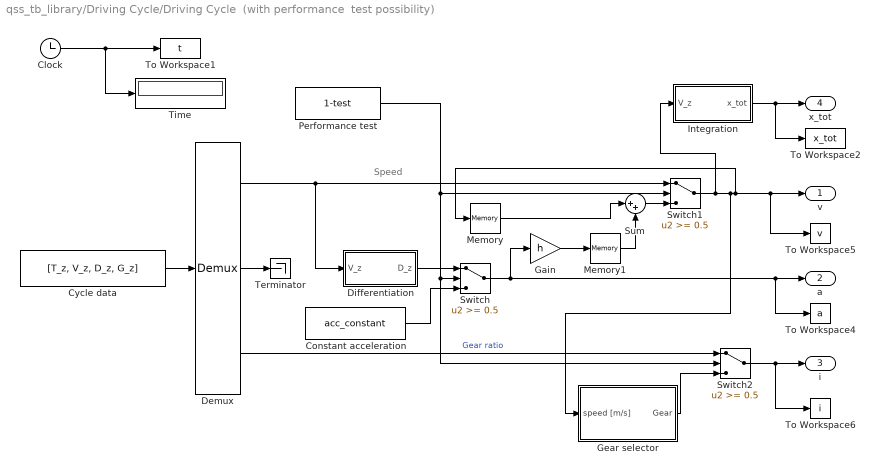
== system qss_tb_library/Driving Cycle/Driving Cycle  (with performance  test possibility) ==
  note: Speed
  Clock : Clock
  Constant acceleration : Constant  Value=acc_constant
  Cycle data : FromWorkspace  VariableName=[T_z, V_z, D_z, G_z]  SampleTime=h
  Demux : Demux  Outputs=3
  Differentiation : Subsystem
  Gain : Gain  Gain=h
  Gear selector : Subsystem
  Integration : Subsystem
  Memory : Memory  InitialCondition=v_init  InheritSampleTime=on
  Memory1 : Memory  InheritSampleTime=on
  Performance test : Constant  Value=1-test
  Sum : Sum  Inputs=|++
  Switch : Switch  Threshold=0.5
  Switch1 : Switch  Threshold=0.5
  Switch2 : Switch  Threshold=0.5
  Terminator : Terminator
  Time : Display
  To Workspace1 : ToWorkspace  VariableName=t  SampleTime=-1
  To Workspace2 : ToWorkspace  VariableName=x_tot  SampleTime=-1
  To Workspace4 : ToWorkspace  VariableName=a  SampleTime=-1
  To Workspace5 : ToWorkspace  VariableName=v  SampleTime=-1
  To Workspace6 : ToWorkspace  VariableName=i  SampleTime=-1
  v : Outport  InitialOutput=0
  a : Outport  Port=2  InitialOutput=0
  i : Outport  Port=3  InitialOutput=0
  x_tot : Outport  Port=4  InitialOutput=0
  wires:
  Clock/1 -> To Workspace1/1, Time/1
  Demux/1 -> Differentiation/1(V_z), Switch1/1
  Demux/2 -> Terminator/1
  Cycle data/1 -> Demux/1
  Differentiation/1(D_z) -> Switch/1
  Switch/1 -> a/1, To Workspace4/1, Gain/1
  Integration/1(x_tot) -> x_tot/1, To Workspace2/1
  Gain/1 -> Memory1/1
  Memory/1 -> Sum/1
  Sum/1 -> Switch1/3
  Constant acceleration/1 -> Switch/3
  Performance test/1 -> Switch1/2, Switch/2, Switch2/2
  Demux/3 -> Switch2/1  "Gear ratio"
  Switch2/1 -> i/1, To Workspace6/1
  Gear selector/1(Gear) -> Switch2/3
  Memory1/1 -> Sum/2
  Switch1/1 -> Integration/1(V_z), v/1, To Workspace5/1, Memory/1, Gear selector/1(speed [m/s])

== system qss_tb_library/Driving Cycle/Driving Cycle (no gradient) ==
  note: Speed
  Clock : Clock
  Cycle data : FromWorkspace  VariableName=[T_z, V_z, D_z, G_z]  SampleTime=h
  Demux : Demux  Outputs=3
  Differentiation : Subsystem
  Integration : Subsystem
  Terminator : Terminator
  Time : Display
  To Workspace1 : ToWorkspace  VariableName=t  SampleTime=-1
  To Workspace2 : ToWorkspace  VariableName=x_tot  SampleTime=-1
  To Workspace4 : ToWorkspace  VariableName=a  SampleTime=-1
  To Workspace5 : ToWorkspace  VariableName=v  SampleTime=-1
  To Workspace6 : ToWorkspace  VariableName=i  SampleTime=-1
  v : Outport  InitialOutput=0
  a : Outport  Port=2  InitialOutput=0
  i : Outport  Port=3  InitialOutput=0
  x_tot : Outport  Port=4  InitialOutput=0
  wires:
  Cycle data/1 -> Demux/1
  Differentiation/1(D_z) -> To Workspace4/1, a/1
  Demux/2 -> Terminator/1
  Integration/1(x_tot) -> x_tot/1, To Workspace2/1
  Demux/3 -> i/1, To Workspace6/1  "Gear ratio"
  Clock/1 -> Time/1, To Workspace1/1
  Demux/1 -> v/1, To Workspace5/1, Integration/1(V_z), Differentiation/1(V_z)

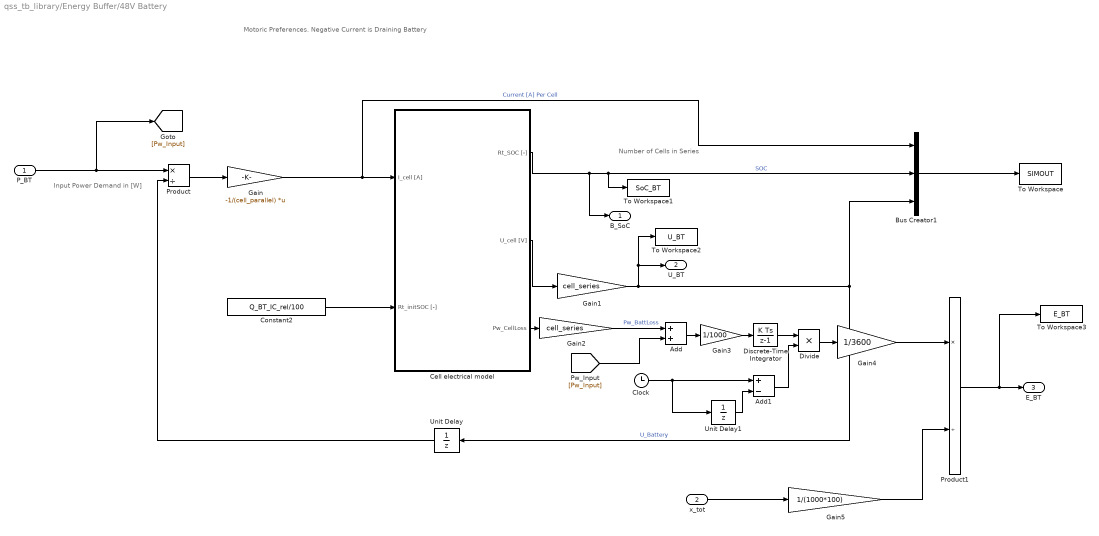
== system qss_tb_library/Energy Buffer/48V Battery ==
  note: Number of Cells in Series
  note: Motoric Preferences. Negative Current is Draining Battery
  note: Input Power Demand in [W]
  P_BT : Inport
  x_tot : Inport  Port=2
  Add : Sum
  Add1 : Sum  Inputs=+-
  Bus Creator1 : BusCreator  Inputs=3
  Cell electrical model : Subsystem
  Clock : Clock
  Constant2 : Constant  Value=Q_BT_IC_rel/100
  Discrete-Time Integrator : DiscreteIntegrator  ICPrevOutput=DiscIntNeverNeededParam  ICPrevScaledInput=DiscIntNeverNeededParam
  Divide : Product  Inputs=**
  Gain : Gain  Gain=-1/(cell_parallel)  Multiplication=Matrix(K*u)
  Gain1 : Gain  Gain=cell_series
  Gain2 : Gain  Gain=cell_series
  Gain3 : Gain  Gain=1/1000
  Gain4 : Gain  Gain=1/3600
  Gain5 : Gain  Gain=1/(1000*100)
  Product : Product  Inputs=*/  RndMeth=Zero
  Product1 : Product  Inputs=*/  SaturateOnIntegerOverflow=on  RndMeth=Zero  InputSameDT=on  OutDataTypeStr=Inherit: Same as first input
  To Workspace : ToWorkspace  VariableName=SIMOUT  SaveFormat=Structure With Time  SampleTime=-1
  To Workspace1 : ToWorkspace  VariableName=SoC_BT  SampleTime=-1
      settings: RequirementInfo={} %GIDa_c6642060_f8db_4366_a618_aa68098668f7
  To Workspace2 : ToWorkspace  VariableName=U_BT  SampleTime=-1
      settings: RequirementInfo={} %GIDa_32590376_96d5_473d_a7bc_23059799ede8
  To Workspace3 : ToWorkspace  VariableName=E_BT  SampleTime=-1
  Unit Delay : UnitDelay  InitialCondition=4.07*cell_series  HasFrameUpgradeWarning=on
  Unit Delay1 : UnitDelay  HasFrameUpgradeWarning=on
  B_SoC : Outport  InitialOutput=0
  U_BT : Outport  Port=2  InitialOutput=0
  E_BT : Outport  Port=3  InitialOutput=0
  wires:
  Add1/1 -> Divide/2
  Unit Delay1/1 -> Add1/2
  Clock/1 -> Add1/1, Unit Delay1/1
  Bus Creator1/1 -> To Workspace/1
  Discrete-Time Integrator/1 -> Divide/1
  x_tot/1 -> Gain5/1
  Gain5/1 -> Product1/2
  Gain4/1 -> Product1/1
  Divide/1 -> Gain4/1
  Gain3/1 -> Discrete-Time Integrator/1
  Add/1 -> Gain3/1
  [Pw_Input] -> Add/2
  Gain2/1 -> Add/1  "Pw_BattLoss"
  Cell electrical model/3(Pw_CellLoss) -> Gain2/1
  Product1/1 -> E_BT/1, To Workspace3/1
  P_BT/1 -> Product/1, [Pw_Input]
  Cell electrical model/1(Rt_SOC [-]) -> Bus Creator1/2, To Workspace1/1, B_SoC/1  "SOC"
  Unit Delay/1 -> Product/2
  Product/1 -> Gain/1
  Constant2/1 -> Cell electrical model/2(Rt_initSOC [-])
  Gain1/1 -> Unit Delay/1, Bus Creator1/3, U_BT/1, To Workspace2/1  "U_Battery"
  Cell electrical model/2(U_cell [V]) -> Gain1/1
  Gain/1 -> Cell electrical model/1(I_cell [A]), Bus Creator1/1  "Current [A] Per Cell"

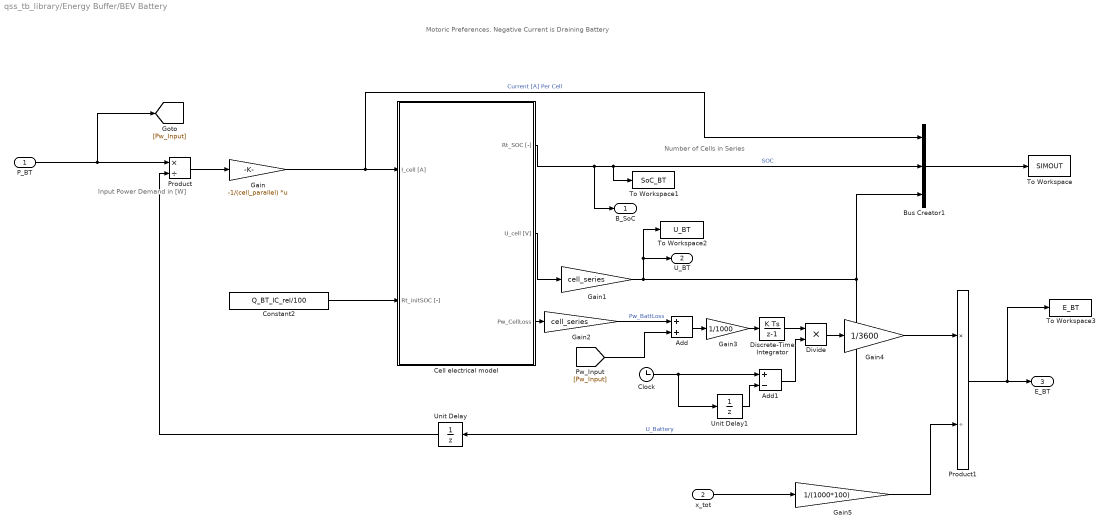
== system qss_tb_library/Energy Buffer/BEV Battery ==
  note: Number of Cells in Series
  note: Motoric Preferences. Negative Current is Draining Battery
  note: Input Power Demand in [W]
  P_BT : Inport
  x_tot : Inport  Port=2
  Add : Sum
  Add1 : Sum  Inputs=+-
  Bus Creator1 : BusCreator  Inputs=3
  Cell electrical model : Subsystem
  Clock : Clock
  Constant2 : Constant  Value=Q_BT_IC_rel/100
  Discrete-Time Integrator : DiscreteIntegrator  ICPrevOutput=DiscIntNeverNeededParam  ICPrevScaledInput=DiscIntNeverNeededParam
  Divide : Product  Inputs=**
  Gain : Gain  Gain=-1/(cell_parallel)  Multiplication=Matrix(K*u)
  Gain1 : Gain  Gain=cell_series
  Gain2 : Gain  Gain=cell_series
  Gain3 : Gain  Gain=1/1000
  Gain4 : Gain  Gain=1/3600
  Gain5 : Gain  Gain=1/(1000*100)
  Product : Product  Inputs=*/  RndMeth=Zero
  Product1 : Product  Inputs=*/  SaturateOnIntegerOverflow=on  RndMeth=Zero  InputSameDT=on  OutDataTypeStr=Inherit: Same as first input
  To Workspace : ToWorkspace  VariableName=SIMOUT  SaveFormat=Structure With Time  SampleTime=-1
  To Workspace1 : ToWorkspace  VariableName=SoC_BT  SampleTime=-1
      settings: RequirementInfo={} %GIDa_c6642060_f8db_4366_a618_aa68098668f7
  To Workspace2 : ToWorkspace  VariableName=U_BT  SampleTime=-1
      settings: RequirementInfo={} %GIDa_32590376_96d5_473d_a7bc_23059799ede8
  To Workspace3 : ToWorkspace  VariableName=E_BT  SampleTime=-1
  Unit Delay : UnitDelay  InitialCondition=4.07*cell_series  HasFrameUpgradeWarning=on
  Unit Delay1 : UnitDelay  HasFrameUpgradeWarning=on
  B_SoC : Outport  InitialOutput=0
  U_BT : Outport  Port=2  InitialOutput=0
  E_BT : Outport  Port=3  InitialOutput=0
  wires:
  Add1/1 -> Divide/2
  Unit Delay1/1 -> Add1/2
  Clock/1 -> Add1/1, Unit Delay1/1
  Bus Creator1/1 -> To Workspace/1
  Discrete-Time Integrator/1 -> Divide/1
  x_tot/1 -> Gain5/1
  Gain5/1 -> Product1/2
  Gain4/1 -> Product1/1
  Divide/1 -> Gain4/1
  Gain3/1 -> Discrete-Time Integrator/1
  Add/1 -> Gain3/1
  [Pw_Input] -> Add/2
  Gain2/1 -> Add/1  "Pw_BattLoss"
  Cell electrical model/3(Pw_CellLoss) -> Gain2/1
  Product1/1 -> E_BT/1, To Workspace3/1
  P_BT/1 -> Product/1, [Pw_Input]
  Cell electrical model/1(Rt_SOC [-]) -> Bus Creator1/2, To Workspace1/1, B_SoC/1  "SOC"
  Unit Delay/1 -> Product/2
  Product/1 -> Gain/1
  Constant2/1 -> Cell electrical model/2(Rt_initSOC [-])
  Gain1/1 -> Unit Delay/1, Bus Creator1/3, U_BT/1, To Workspace2/1  "U_Battery"
  Cell electrical model/2(U_cell [V]) -> Gain1/1
  Gain/1 -> Cell electrical model/1(I_cell [A]), Bus Creator1/1  "Current [A] Per Cell"

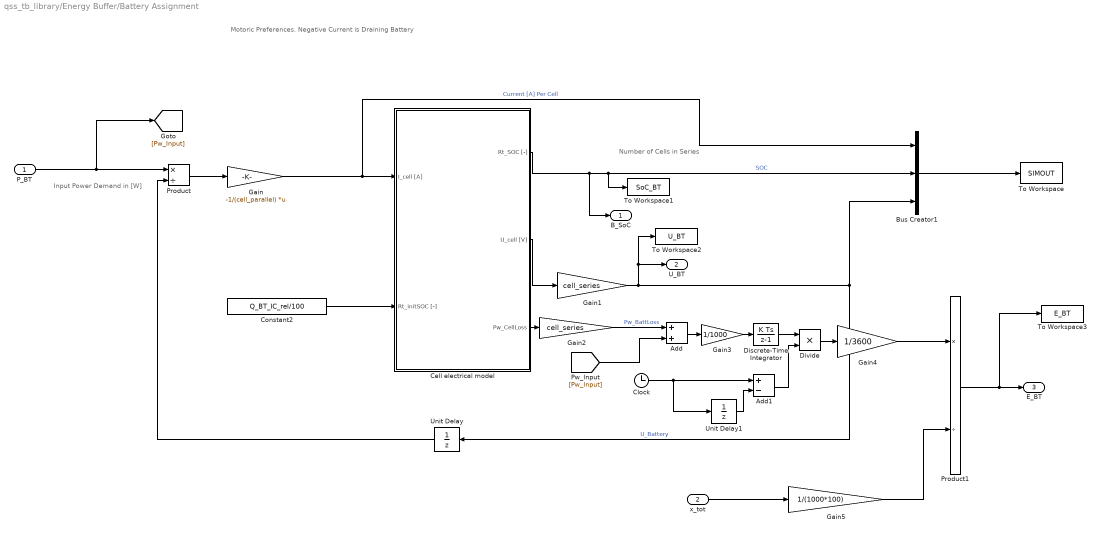
== system qss_tb_library/Energy Buffer/Battery Assignment ==
  note: Number of Cells in Series
  note: Motoric Preferences. Negative Current is Draining Battery
  note: Input Power Demand in [W]
  P_BT : Inport
  x_tot : Inport  Port=2
  Add : Sum
  Add1 : Sum  Inputs=+-
  Bus Creator1 : BusCreator  Inputs=3
  Cell electrical model : Subsystem
  Clock : Clock
  Constant2 : Constant  Value=Q_BT_IC_rel/100
  Discrete-Time Integrator : DiscreteIntegrator  ICPrevOutput=DiscIntNeverNeededParam  ICPrevScaledInput=DiscIntNeverNeededParam
  Divide : Product  Inputs=**
  Gain : Gain  Gain=-1/(cell_parallel)  Multiplication=Matrix(K*u)
  Gain1 : Gain  Gain=cell_series
  Gain2 : Gain  Gain=cell_series
  Gain3 : Gain  Gain=1/1000
  Gain4 : Gain  Gain=1/3600
  Gain5 : Gain  Gain=1/(1000*100)
  Product : Product  Inputs=*/  RndMeth=Zero
  Product1 : Product  Inputs=*/  SaturateOnIntegerOverflow=on  RndMeth=Zero  InputSameDT=on  OutDataTypeStr=Inherit: Same as first input
  To Workspace : ToWorkspace  VariableName=SIMOUT  SaveFormat=Structure With Time  SampleTime=-1
  To Workspace1 : ToWorkspace  VariableName=SoC_BT  SampleTime=-1
      settings: RequirementInfo={} %GIDa_c6642060_f8db_4366_a618_aa68098668f7
  To Workspace2 : ToWorkspace  VariableName=U_BT  SampleTime=-1
      settings: RequirementInfo={} %GIDa_32590376_96d5_473d_a7bc_23059799ede8
  To Workspace3 : ToWorkspace  VariableName=E_BT  SampleTime=-1
  Unit Delay : UnitDelay  InitialCondition=4.07*cell_series  HasFrameUpgradeWarning=on
  Unit Delay1 : UnitDelay  HasFrameUpgradeWarning=on
  B_SoC : Outport  InitialOutput=0
  U_BT : Outport  Port=2  InitialOutput=0
  E_BT : Outport  Port=3  InitialOutput=0
  wires:
  Add1/1 -> Divide/2
  Unit Delay1/1 -> Add1/2
  Clock/1 -> Add1/1, Unit Delay1/1
  Bus Creator1/1 -> To Workspace/1
  Discrete-Time Integrator/1 -> Divide/1
  x_tot/1 -> Gain5/1
  Gain5/1 -> Product1/2
  Gain4/1 -> Product1/1
  Divide/1 -> Gain4/1
  Gain3/1 -> Discrete-Time Integrator/1
  Add/1 -> Gain3/1
  [Pw_Input] -> Add/2
  Gain2/1 -> Add/1  "Pw_BattLoss"
  Cell electrical model/3(Pw_CellLoss) -> Gain2/1
  Product1/1 -> E_BT/1, To Workspace3/1
  P_BT/1 -> Product/1, [Pw_Input]
  Cell electrical model/1(Rt_SOC [-]) -> Bus Creator1/2, To Workspace1/1, B_SoC/1  "SOC"
  Unit Delay/1 -> Product/2
  Product/1 -> Gain/1
  Constant2/1 -> Cell electrical model/2(Rt_initSOC [-])
  Gain1/1 -> Unit Delay/1, Bus Creator1/3, U_BT/1, To Workspace2/1  "U_Battery"
  Cell electrical model/2(U_cell [V]) -> Gain1/1
  Gain/1 -> Cell electrical model/1(I_cell [A]), Bus Creator1/1  "Current [A] Per Cell"

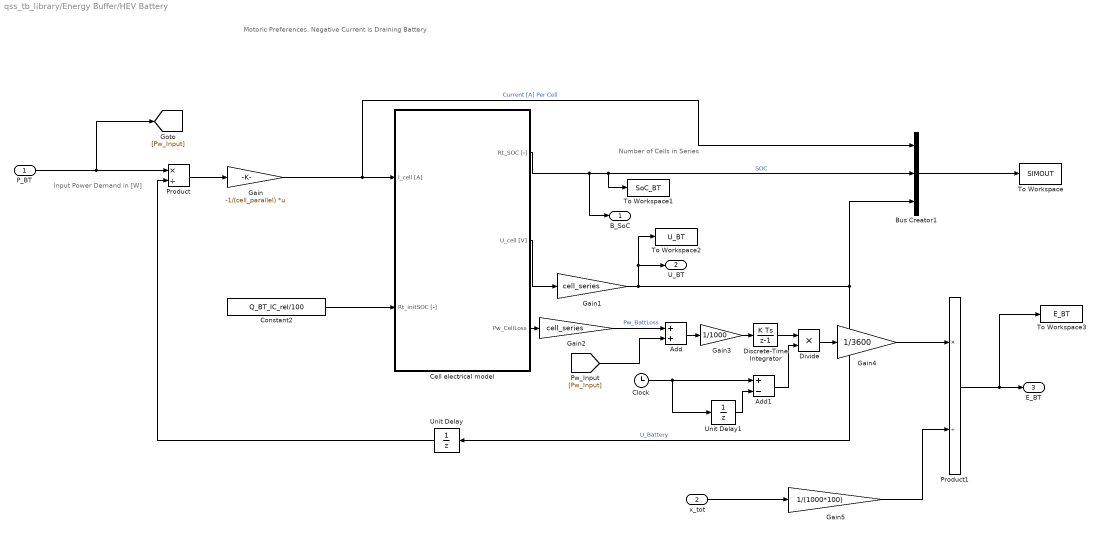
== system qss_tb_library/Energy Buffer/HEV Battery ==
  note: Number of Cells in Series
  note: Motoric Preferences. Negative Current is Draining Battery
  note: Input Power Demand in [W]
  P_BT : Inport
  x_tot : Inport  Port=2
  Add : Sum
  Add1 : Sum  Inputs=+-
  Bus Creator1 : BusCreator  Inputs=3
  Cell electrical model : Subsystem
  Clock : Clock
  Constant2 : Constant  Value=Q_BT_IC_rel/100
  Discrete-Time Integrator : DiscreteIntegrator  ICPrevOutput=DiscIntNeverNeededParam  ICPrevScaledInput=DiscIntNeverNeededParam
  Divide : Product  Inputs=**
  Gain : Gain  Gain=-1/(cell_parallel)  Multiplication=Matrix(K*u)
  Gain1 : Gain  Gain=cell_series
  Gain2 : Gain  Gain=cell_series
  Gain3 : Gain  Gain=1/1000
  Gain4 : Gain  Gain=1/3600
  Gain5 : Gain  Gain=1/(1000*100)
  Product : Product  Inputs=*/  RndMeth=Zero
  Product1 : Product  Inputs=*/  SaturateOnIntegerOverflow=on  RndMeth=Zero  InputSameDT=on  OutDataTypeStr=Inherit: Same as first input
  To Workspace : ToWorkspace  VariableName=SIMOUT  SaveFormat=Structure With Time  SampleTime=-1
  To Workspace1 : ToWorkspace  VariableName=SoC_BT  SampleTime=-1
      settings: RequirementInfo={} %GIDa_c6642060_f8db_4366_a618_aa68098668f7
  To Workspace2 : ToWorkspace  VariableName=U_BT  SampleTime=-1
      settings: RequirementInfo={} %GIDa_32590376_96d5_473d_a7bc_23059799ede8
  To Workspace3 : ToWorkspace  VariableName=E_BT  SampleTime=-1
  Unit Delay : UnitDelay  InitialCondition=4.07*cell_series  HasFrameUpgradeWarning=on
  Unit Delay1 : UnitDelay  HasFrameUpgradeWarning=on
  B_SoC : Outport  InitialOutput=0
  U_BT : Outport  Port=2  InitialOutput=0
  E_BT : Outport  Port=3  InitialOutput=0
  wires:
  Add1/1 -> Divide/2
  Unit Delay1/1 -> Add1/2
  Clock/1 -> Add1/1, Unit Delay1/1
  Bus Creator1/1 -> To Workspace/1
  Discrete-Time Integrator/1 -> Divide/1
  x_tot/1 -> Gain5/1
  Gain5/1 -> Product1/2
  Gain4/1 -> Product1/1
  Divide/1 -> Gain4/1
  Gain3/1 -> Discrete-Time Integrator/1
  Add/1 -> Gain3/1
  [Pw_Input] -> Add/2
  Gain2/1 -> Add/1  "Pw_BattLoss"
  Cell electrical model/3(Pw_CellLoss) -> Gain2/1
  Product1/1 -> E_BT/1, To Workspace3/1
  P_BT/1 -> Product/1, [Pw_Input]
  Cell electrical model/1(Rt_SOC [-]) -> Bus Creator1/2, To Workspace1/1, B_SoC/1  "SOC"
  Unit Delay/1 -> Product/2
  Product/1 -> Gain/1
  Constant2/1 -> Cell electrical model/2(Rt_initSOC [-])
  Gain1/1 -> Unit Delay/1, Bus Creator1/3, U_BT/1, To Workspace2/1  "U_Battery"
  Cell electrical model/2(U_cell [V]) -> Gain1/1
  Gain/1 -> Cell electrical model/1(I_cell [A]), Bus Creator1/1  "Current [A] Per Cell"
